simulink model "ACStesbed1"  (R2013b)
settings: Solver=ode45  StartTime=0.0  StopTime=10000  FixedStep=0.01  RelTol=1e-3
StartFcn:
  | InitializeModel
undefined symbols (not defined in the file or in its folder): DiscIntNeverNeededParam, e0_0, e1_0, e2_0, e3_0, magnitude, OrbData, params
libraries: aerolibutil x29, vrlib x26, satellite_control_lib x17, aerolibtransform2 x5, dspmtrx3 x5, aerolib6dofsys x4, dspinverses x3, simulink x3, aerolib6dof2 x1
(part 2 of 2)

== system ACStesbed1/CentralComputer/SatAttitude/BINS/OrbitalBasis ==
  vj2000 : Inport
  rj2000 : Inport  Port=2
  Cross Product : vrlib/Utilities/Cross Product
  Cross Product1 : vrlib/Utilities/Cross Product
  Direction Cosine Matrix to Quaternions : aerolibtransform2/Direction Cosine Matrix  to Quaternions
  Display4 : Display
  Divide : Product  Inputs=*/
  Gain : Gain  Gain=-1
  Matrix Concatenate : Concatenate  NumInputs=3  Mode=Multidimensional array  ConcatenateDimension=2
  Normalize Vector : vrlib/Utilities/Normalize Vector  maxzero=0.00001
  Normalize Vector1 : vrlib/Utilities/Normalize Vector  maxzero=0.00001
  Signal Specification : SignalSpecification  Dimensions=3
  Signal Specification1 : SignalSpecification  Dimensions=3
  Transpose1 : dspmtrx3/Transpose  Hermitian=off  overflowFlag=off
  vectnorm : Fcn  Expr=u(1)^2+u(2)^2+u(3)^2
  Qjo : Outport
  Worb_j : Outport  Port=2
  wires:
  Cross Product1/1 -> Signal Specification1/1  "iorb"
  Normalize Vector/1 -> Matrix Concatenate/2, Cross Product1/1  "jorb"
  Matrix Concatenate/1 -> Transpose1/1  "DCMoj"
  rj2000/1 -> Cross Product/2, Normalize Vector/1, vectnorm/1
  vj2000/1 -> Cross Product/1
  Direction Cosine Matrix to Quaternions/1 -> Display4/1, Qjo/1  "Qjo"
  Normalize Vector1/1 -> Matrix Concatenate/3, Cross Product1/2  "korb"
  Cross Product/1 -> Signal Specification/1
  Gain/1 -> Divide/1
  vectnorm/1 -> Divide/2
  Divide/1 -> Worb_j/1
  Signal Specification/1 -> Gain/1, Normalize Vector1/1
  Signal Specification1/1 -> Matrix Concatenate/1
  Transpose1/1 -> Direction Cosine Matrix to Quaternions/1  "DCMjo"

== system ACStesbed1/CentralComputer/SatAttitude/BINS/SIgnQuat ==
  Q : Inport
  Product : Product
  Selector2 : Selector  InputPortWidth=4  IndexOptions=Index vector (dialog)  Indices=[1]  OutputSizes=1
  Sign : Signum
  Q' : Outport
  wires:
  Q/1 -> Product/2, Selector2/1
  Product/1 -> Q'/1
  Sign/1 -> Product/1
  Selector2/1 -> Sign/1

== system ACStesbed1/CentralComputer/SatAttitude/BINS/SIgnQuat1 ==
  Q : Inport
  Constant : Constant
  Constant1 : Constant  Value=-1
  Product : Product
  Selector2 : Selector  InputPortWidth=4  IndexOptions=Index vector (dialog)  Indices=[1]  OutputSizes=1
  Switch : Switch
  Q' : Outport
  wires:
  Q/1 -> Product/2, Selector2/1
  Product/1 -> Q'/1
  Switch/1 -> Product/1
  Selector2/1 -> Switch/2
  Constant/1 -> Switch/1
  Constant1/1 -> Switch/3

== system ACStesbed1/CentralComputer/SatAttitude/BINS/SIgnQuat2 ==
  Q : Inport
  Constant : Constant
  Constant1 : Constant  Value=-1
  Product : Product
  Selector2 : Selector  InputPortWidth=4  IndexOptions=Index vector (dialog)  Indices=[1]  OutputSizes=1
  Switch : Switch
  Q' : Outport
  wires:
  Q/1 -> Product/2, Selector2/1
  Product/1 -> Q'/1
  Switch/1 -> Product/1
  Selector2/1 -> Switch/2
  Constant/1 -> Switch/1
  Constant1/1 -> Switch/3

== system ACStesbed1/CentralComputer/SatAttitude/BINS/SIgnQuat3 ==
  Q : Inport
  Constant : Constant
  Constant1 : Constant  Value=-1
  Product : Product
  Selector2 : Selector  InputPortWidth=4  IndexOptions=Index vector (dialog)  Indices=[1]  OutputSizes=1
  Switch : Switch
  Q' : Outport
  wires:
  Q/1 -> Product/2, Selector2/1
  Product/1 -> Q'/1
  Switch/1 -> Product/1
  Selector2/1 -> Switch/2
  Constant/1 -> Switch/1
  Constant1/1 -> Switch/3

== system ACStesbed1/CentralComputer/SatAttitude/BINS/SIgnQuat4 ==
  Q : Inport
  Constant : Constant
  Constant1 : Constant  Value=-1
  Product : Product
  Selector2 : Selector  InputPortWidth=4  IndexOptions=Index vector (dialog)  Indices=[1]  OutputSizes=1
  Switch : Switch
  Q' : Outport
  wires:
  Q/1 -> Product/2, Selector2/1
  Product/1 -> Q'/1
  Switch/1 -> Product/1
  Selector2/1 -> Switch/2
  Constant/1 -> Switch/1
  Constant1/1 -> Switch/3

== system ACStesbed1/CentralComputer/SatAttitude/BINS/quatint ==
  p q r : Inport
  q_init : Inport  Port=2
  q0 q1 q2 q3 : Integrator  InitialConditionSource=external  InitialCondition=[e0_0 e1_0 e2_0 e3_0]
  qdot : aerolib6dofsys/DCM & Euler Angles (Quaternion)/qdot
  q : Outport
  wires:
  q0 q1 q2 q3/1 -> q/1, qdot/2
  q_init/1 -> q0 q1 q2 q3/2
  p q r/1 -> qdot/1
  qdot/1 -> q0 q1 q2 q3/1

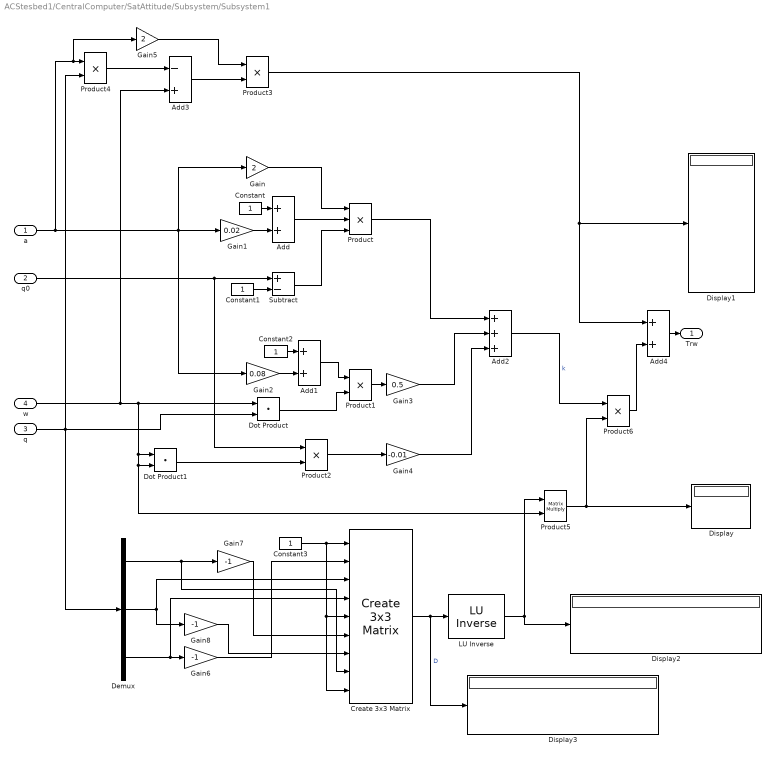
== system ACStesbed1/CentralComputer/SatAttitude/Subsystem/Subsystem1 ==
  a : Inport
  q0 : Inport  Port=2
  q : Inport  Port=3
  w : Inport  Port=4
  " LU Inverse" : dspinverses/ LU Inverse
  Add : Sum
  Add1 : Sum
  Add2 : Sum  Inputs=+++
  Add3 : Sum  Inputs=-+
  Add4 : Sum
  Constant{,1..3} (4 alike) : Constant
  Create 3x3 Matrix : aerolibutil/Create 3x3 Matrix
  Demux : Demux  Outputs=3
  Display{,1..3} (4 alike) : Display
  Dot Product : DotProduct  InputSameDT=on  OutDataTypeStr=Inherit: Inherit via internal rule
  Dot Product1 : DotProduct  InputSameDT=on  OutDataTypeStr=Inherit: Inherit via internal rule
  Gain : Gain  Gain=2
  Gain1 : Gain  Gain=0.02
  Gain2 : Gain  Gain=0.08
  Gain3 : Gain  Gain=0.5
  Gain4 : Gain  Gain=-0.01
  Gain5 : Gain  Gain=2
  Gain6 : Gain  Gain=-1
  Gain7 : Gain  Gain=-1
  Gain8 : Gain  Gain=-1
  Product : Product  Inputs=3
  Product{1..4,6} (5 alike) : Product
  Product5 : Product  Multiplication=Matrix(*)
  Subtract : Sum  Inputs=+-
  Trw : Outport
  wires:
  Gain1/1 -> Add/2
  Constant/1 -> Add/1
  a/1 -> Gain5/1, Product4/1, Gain2/1, Gain/1, Gain1/1
  Constant1/1 -> Subtract/2
  q0/1 -> Product2/1, Subtract/1
  Gain/1 -> Product/1
  Add/1 -> Product/2
  Subtract/1 -> Product/3
  w/1 -> Add3/2, Dot Product/1, Product5/2, Dot Product1/2, Dot Product1/1
  q/1 -> Demux/1, Product4/2, Dot Product/2
  Gain2/1 -> Add1/2
  Constant2/1 -> Add1/1
  Add1/1 -> Product1/1
  Dot Product/1 -> Product1/2
  Product1/1 -> Gain3/1
  Dot Product1/1 -> Product2/2
  Product2/1 -> Gain4/1
  Product/1 -> Add2/1
  Gain3/1 -> Add2/2
  Gain4/1 -> Add2/3
  Add2/1 -> Product6/1  "k"
  Product4/1 -> Add3/1
  Gain5/1 -> Product3/1
  Add3/1 -> Product3/2
  Constant3/1 -> Create 3x3 Matrix/9, Create 3x3 Matrix/5, Create 3x3 Matrix/1
  Demux/3 -> Create 3x3 Matrix/4, Gain6/1
  Gain6/1 -> Create 3x3 Matrix/2
  Demux/2 -> Gain8/1, Create 3x3 Matrix/3
  Demux/1 -> Create 3x3 Matrix/8, Gain7/1
  Gain7/1 -> Create 3x3 Matrix/6
  Gain8/1 -> Create 3x3 Matrix/7
  Create 3x3 Matrix/1 -> Display3/1, " LU Inverse"/1  "D"
  " LU Inverse"/1 -> Product5/1, Display2/1
  Product5/1 -> Display/1, Product6/2
  Add4/1 -> Trw/1
  Product6/1 -> Add4/2
  Product3/1 -> Display1/1, Add4/1

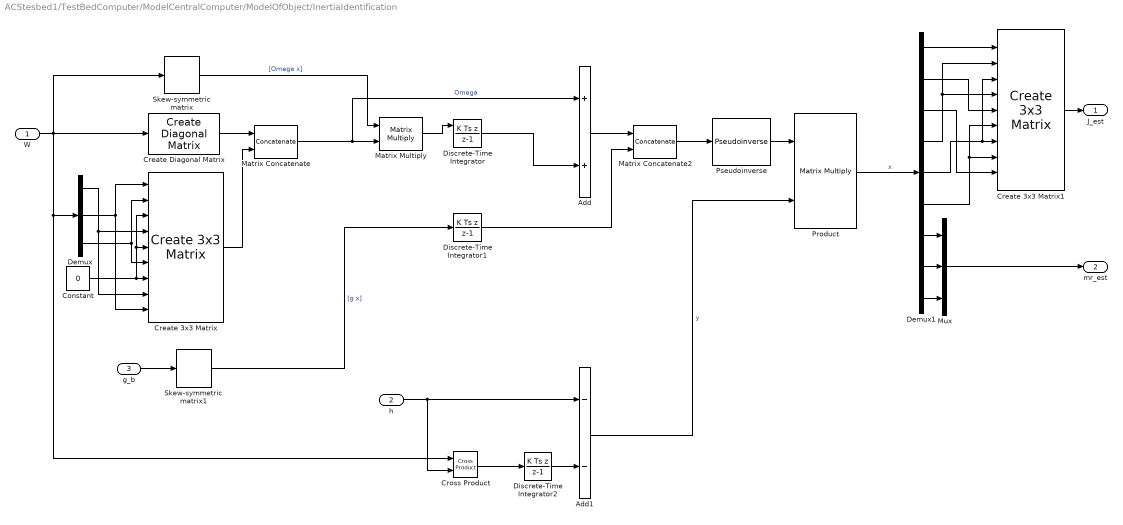
== system ACStesbed1/TestBedComputer/ModelCentralComputer/ModelOfObject/InertiaIdentification ==
  W : Inport
  h : Inport  Port=2
  g_b : Inport  Port=3
  Add : Sum
  Add1 : Sum  Inputs=--
  Constant : Constant  Value=0
  Create 3x3 Matrix : aerolibutil/Create 3x3 Matrix
  Create 3x3 Matrix1 : aerolibutil/Create 3x3 Matrix
  Create Diagonal Matrix : dspmtrx3/Create Diagonal Matrix
  Cross Product : vrlib/Utilities/Cross Product
  Demux : Demux  Outputs=3
  Demux1 : Demux  Outputs=9
  Discrete-Time Integrator : DiscreteIntegrator  IntegratorMethod=Integration: Backward Euler  InitialConditionSource=external  ICPrevOutput=DiscIntNeverNeededParam  ICPrevScaledInput=DiscIntNeverNeededParam
  Discrete-Time Integrator1 : DiscreteIntegrator  IntegratorMethod=Integration: Backward Euler  ICPrevOutput=DiscIntNeverNeededParam  ICPrevScaledInput=DiscIntNeverNeededParam
  Discrete-Time Integrator2 : DiscreteIntegrator  IntegratorMethod=Integration: Backward Euler  ICPrevOutput=DiscIntNeverNeededParam  ICPrevScaledInput=DiscIntNeverNeededParam
  Matrix Concatenate : Concatenate  Mode=Multidimensional array  ConcatenateDimension=2
  Matrix Concatenate2 : Concatenate  Mode=Multidimensional array  ConcatenateDimension=2
  Matrix Multiply : Product  Multiplication=Matrix(*)
  Mux : Mux  Inputs=3
  Product : Product  Multiplication=Matrix(*)
  Pseudoinverse : dspinverses/Pseudoinverse  wanterr=off
  Skew-symmetric matrix : satellite_control_lib/Skew-symmetric matrix
  Skew-symmetric matrix1 : satellite_control_lib/Skew-symmetric matrix
  J_est : Outport
  mr_est : Outport  Port=2
  wires:
  Product/1 -> Demux1/1  "x"
  Pseudoinverse/1 -> Product/1
  Add1/1 -> Product/2  "y"
  W/1 -> Skew-symmetric matrix/1, Demux/1, Cross Product/1, Create Diagonal Matrix/1
  Demux/2 -> Create 3x3 Matrix/9, Create 3x3 Matrix/1
  Demux/3 -> Create 3x3 Matrix/6, Create 3x3 Matrix/2
  Demux/1 -> Create 3x3 Matrix/8, Create 3x3 Matrix/4
  Constant/1 -> Create 3x3 Matrix/3, Create 3x3 Matrix/5, Create 3x3 Matrix/7
  Create Diagonal Matrix/1 -> Matrix Concatenate/1
  Create 3x3 Matrix/1 -> Matrix Concatenate/2
  Matrix Concatenate/1 -> Add/1, Matrix Multiply/2  "Omega"
  Skew-symmetric matrix/1 -> Matrix Multiply/1  "[Omega x]"
  g_b/1 -> Skew-symmetric matrix1/1
  Skew-symmetric matrix1/1 -> Discrete-Time Integrator1/1  "[g x]"
  Matrix Multiply/1 -> Discrete-Time Integrator/1
  Discrete-Time Integrator1/1 -> Matrix Concatenate2/2
  Discrete-Time Integrator/1 -> Add/2
  Add/1 -> Matrix Concatenate2/1
  h/1 -> Cross Product/2, Add1/1
  Discrete-Time Integrator2/1 -> Add1/2
  Cross Product/1 -> Discrete-Time Integrator2/1
  Demux1/1 -> Create 3x3 Matrix1/1
  Demux1/2 -> Create 3x3 Matrix1/5
  Demux1/3 -> Create 3x3 Matrix1/9
  Demux1/4 -> Create 3x3 Matrix1/4, Create 3x3 Matrix1/2
  Demux1/5 -> Create 3x3 Matrix1/7, Create 3x3 Matrix1/3
  Demux1/6 -> Create 3x3 Matrix1/8, Create 3x3 Matrix1/6
  Create 3x3 Matrix1/1 -> J_est/1
  Demux1/7 -> Mux/1
  Demux1/9 -> Mux/3
  Demux1/8 -> Mux/2
  Mux/1 -> mr_est/1
  Matrix Concatenate2/1 -> Pseudoinverse/1

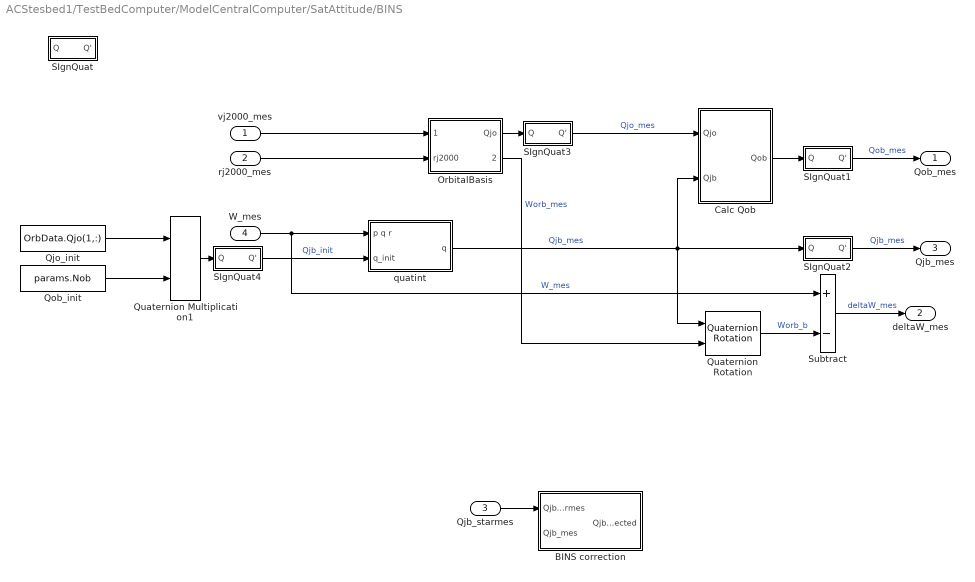
== system ACStesbed1/TestBedComputer/ModelCentralComputer/SatAttitude/BINS ==
  vj2000_mes : Inport
  rj2000_mes : Inport  Port=2
  Qjb_starmes : Inport  Port=3
  W_mes : Inport  Port=4
  BINS correction : Subsystem
  Calc Qob : Subsystem
  OrbitalBasis : Subsystem
  Qjo_init : Constant  Value=OrbData.Qjo(1,:)
  Qob_init : Constant  Value=params.Nob
  Quaternion Multiplication1 : aerolibutil/Quaternion Multiplication
  Quaternion Rotation : aerolibutil/Quaternion Rotation
  SIgnQuat : Subsystem
  SIgnQuat1 : Subsystem
  SIgnQuat2 : Subsystem
  SIgnQuat3 : Subsystem
  SIgnQuat4 : Subsystem
  Subtract : Sum  Inputs=+-
  quatint : Subsystem
  Qob_mes : Outport
  deltaW_mes : Outport  Port=2
  Qjb_mes : Outport  Port=3
  wires:
  Qjb_starmes/1 -> BINS correction/1(Qjb_starmes)
  quatint/1(q) -> SIgnQuat2/1(Q), Calc Qob/2(Qjb), Quaternion Rotation/1  "Qjb_mes"
  Calc Qob/1(Qob) -> SIgnQuat1/1(Q)
  rj2000_mes/1 -> OrbitalBasis/2(rj2000)
  vj2000_mes/1 -> OrbitalBasis/1(vj2000)
  OrbitalBasis/1(Qjo) -> SIgnQuat3/1(Q)
  OrbitalBasis/2(Worb_j) -> Quaternion Rotation/2  "Worb_mes"
  W_mes/1 -> Subtract/1, quatint/1(p q r)  "W_mes"
  Subtract/1 -> deltaW_mes/1  "deltaW_mes"
  Qjo_init/1 -> Quaternion Multiplication1/1
  Qob_init/1 -> Quaternion Multiplication1/2
  Quaternion Multiplication1/1 -> SIgnQuat4/1(Q)
  Quaternion Rotation/1 -> Subtract/2  "Worb_b"
  SIgnQuat1/1(Q') -> Qob_mes/1  "Qob_mes"
  SIgnQuat2/1(Q') -> Qjb_mes/1  "Qjb_mes"
  SIgnQuat3/1(Q') -> Calc Qob/1(Qjo)  "Qjo_mes"
  SIgnQuat4/1(Q') -> quatint/2(q_init)  "Qjb_init"

== system ACStesbed1/TestBedComputer/ModelCentralComputer/SatAttitude/Subsystem ==
  In1 : Inport
  In2 : Inport  Port=2
  In3 : Inport  Port=3
  Gain : Gain  Gain=-1
  Product5 : Product  Multiplication=Matrix(*)
  Selector : Selector  InputPortWidth=4  IndexOptions=Index vector (dialog)  Indices=1  OutputSizes=1
  Selector1 : Selector  InputPortWidth=4  IndexOptions=Index vector (dialog)  Indices=[2 3 4]  OutputSizes=1
  Subsystem1 : Subsystem
  a : Constant  Value=-0.9
  Out1 : Outport
  wires:
  Subsystem1/1(Trw) -> Product5/2
  Selector1/1 -> Subsystem1/3(q)
  a/1 -> Subsystem1/1(a)
  Selector/1 -> Subsystem1/2(q0)  "1"
  Product5/1 -> Gain/1
  In2/1 -> Selector1/1, Selector/1
  In3/1 -> Subsystem1/4(w)
  In1/1 -> Product5/1
  Gain/1 -> Out1/1

== system ACStesbed1/TestBedComputer/ModelObject/Inertia/deltaJ1 ==
  d : Inport
  e : Inport  Port=2
  rho : Inport  Port=3
  Add : Sum  Inputs=3
  Constant : Constant  Value=params.bmass
  Gain : Gain  Gain=-1
  Math Function : Math  Operator=magnitude^2  SaturateOnIntegerOverflow=on
  Product{,4..6} (4 alike) : Product
  Product1 : Product  Multiplication=Matrix(*)
  Product2 : Product  Multiplication=Matrix(*)
  Product3 : Product  Multiplication=Matrix(*)
  Skew-symmetric matrix : satellite_control_lib/Skew-symmetric matrix
  Skew-symmetric matrix1 : satellite_control_lib/Skew-symmetric matrix
  deltaJ : Outport
  wires:
  Constant/1 -> Gain/1
  e/1 -> Skew-symmetric matrix/1
  rho/1 -> Skew-symmetric matrix1/1
  Product/1 -> deltaJ/1  "(-m)(d^2[e x]^2+d[rho x][e x]+d[e x][rho x])"
  Gain/1 -> Product/1
  d/1 -> Math Function/1, Product6/1, Product5/1
  Skew-symmetric matrix/1 -> Product2/2, Product3/1, Product1/1, Product1/2  "[e x]"
  Math Function/1 -> Product4/1
  Product1/1 -> Product4/2
  Skew-symmetric matrix1/1 -> Product3/2, Product2/1  "[rho x]"
  Product3/1 -> Product5/2
  Product2/1 -> Product6/2
  Add/1 -> Product/2
  Product4/1 -> Add/1
  Product5/1 -> Add/2
  Product6/1 -> Add/3

== system ACStesbed1/TestBedComputer/ModelObject/Inertia/deltaJ2 ==
  d : Inport
  e : Inport  Port=2
  rho : Inport  Port=3
  Add : Sum  Inputs=3
  Constant : Constant  Value=params.bmass
  Gain : Gain  Gain=-1
  Math Function : Math  Operator=magnitude^2  SaturateOnIntegerOverflow=on
  Product{,4..6} (4 alike) : Product
  Product1 : Product  Multiplication=Matrix(*)
  Product2 : Product  Multiplication=Matrix(*)
  Product3 : Product  Multiplication=Matrix(*)
  Skew-symmetric matrix : satellite_control_lib/Skew-symmetric matrix
  Skew-symmetric matrix1 : satellite_control_lib/Skew-symmetric matrix
  deltaJ : Outport
  wires:
  Product6/1 -> Add/3
  Product5/1 -> Add/2
  Product4/1 -> Add/1
  Add/1 -> Product/2
  Product2/1 -> Product6/2
  Product3/1 -> Product5/2
  Skew-symmetric matrix1/1 -> Product2/1, Product3/2  "[rho x]"
  Product1/1 -> Product4/2
  Math Function/1 -> Product4/1
  Skew-symmetric matrix/1 -> Product1/2, Product1/1, Product3/1, Product2/2  "[e x]"
  d/1 -> Product5/1, Product6/1, Math Function/1
  Gain/1 -> Product/1
  Product/1 -> deltaJ/1  "(-m)(d^2[e x]^2+d[rho x][e x]+d[e x][rho x])"
  rho/1 -> Skew-symmetric matrix1/1
  e/1 -> Skew-symmetric matrix/1
  Constant/1 -> Gain/1

== system ACStesbed1/TestBedComputer/ModelObject/Inertia/deltaJ3 ==
  d : Inport
  e : Inport  Port=2
  rho : Inport  Port=3
  Add : Sum  Inputs=3
  Constant : Constant  Value=params.bmass
  Gain : Gain  Gain=-1
  Math Function : Math  Operator=magnitude^2  SaturateOnIntegerOverflow=on
  Product{,4..6} (4 alike) : Product
  Product1 : Product  Multiplication=Matrix(*)
  Product2 : Product  Multiplication=Matrix(*)
  Product3 : Product  Multiplication=Matrix(*)
  Skew-symmetric matrix : satellite_control_lib/Skew-symmetric matrix
  Skew-symmetric matrix1 : satellite_control_lib/Skew-symmetric matrix
  deltaJ : Outport
  wires:
  Constant/1 -> Gain/1
  e/1 -> Skew-symmetric matrix/1
  rho/1 -> Skew-symmetric matrix1/1
  Product/1 -> deltaJ/1  "(-m)(d^2[e x]^2+d[rho x][e x]+d[e x][rho x])"
  Gain/1 -> Product/1
  d/1 -> Math Function/1, Product6/1, Product5/1
  Skew-symmetric matrix/1 -> Product2/2, Product3/1, Product1/1, Product1/2  "[e x]"
  Math Function/1 -> Product4/1
  Product1/1 -> Product4/2
  Skew-symmetric matrix1/1 -> Product3/2, Product2/1  "[rho x]"
  Product3/1 -> Product5/2
  Product2/1 -> Product6/2
  Add/1 -> Product/2
  Product4/1 -> Add/1
  Product5/1 -> Add/2
  Product6/1 -> Add/3

== system ACStesbed1/TestBedComputer/ModelObject/TestBedDynamics/quatint ==
  p q r : Inport
  q_init : Inport  Port=2
  Discrete-Time Integrator : DiscreteIntegrator  InitialConditionSource=external  ICPrevOutput=DiscIntNeverNeededParam  ICPrevScaledInput=DiscIntNeverNeededParam
  qdot : aerolib6dofsys/DCM & Euler Angles (Quaternion)/qdot
  q : Outport
  wires:
  Discrete-Time Integrator/1 -> q/1, qdot/2
  q_init/1 -> Discrete-Time Integrator/2
  p q r/1 -> qdot/1
  qdot/1 -> Discrete-Time Integrator/1

== system ACStesbed1/TestBedComputer/ModelObject/Torques/Tm ==
  L : Inport
  B : Inport  Port=2
  Ldisturb : Inport  Port=3
  Tm : Outport
  wires:
  L/1 -> Tm/1

== system ACStesbed1/TestBedComputer/ModelObject/Torques/Tothers ==
  Something : Inport
  Tothers : Outport
  wires:
  Something/1 -> Tothers/1

== system ACStesbed1/TestBedComputer/ModelObject/Torques/Trw ==
  dh : Inport
  W : Inport  Port=2
  h : Inport  Port=3
  Add : Sum
  Cross Product : vrlib/Utilities/Cross Product
  Gain : Gain  Gain=-1
  Trw : Outport
  wires:
  W/1 -> Cross Product/1
  Gain/1 -> Trw/1  "Trw"
  Cross Product/1 -> Add/2  "Wxh"
  Add/1 -> Gain/1  "(dH+WxH)"
  dh/1 -> Add/1
  h/1 -> Cross Product/2

== system ACStesbed1/TestBedComputer/ModelCentralComputer/SatAttitude/BINS/BINS correction ==
  Qjb_starmes : Inport
  Qjb_mes : Inport  Port=2
  Quaternion Conjugate : aerolibutil/Quaternion Conjugate
  Quaternion Conjugate1 : aerolibutil/Quaternion Conjugate
  Quaternion Multiplication : aerolibutil/Quaternion Multiplication
  Quaternion Multiplication1 : aerolibutil/Quaternion Multiplication
  Qjb_corrected : Outport
  wires:
  Quaternion Multiplication1/1 -> Qjb_corrected/1  "Qjb_corrected"
  Quaternion Conjugate1/1 -> Quaternion Multiplication1/1
  Qjb_mes/1 -> Quaternion Multiplication1/2, Quaternion Multiplication/2
  Quaternion Multiplication/1 -> Quaternion Conjugate1/1  "Nbb_mes"
  Qjb_starmes/1 -> Quaternion Conjugate/1
  Quaternion Conjugate/1 -> Quaternion Multiplication/1  "conjQjb_starmes"

== system ACStesbed1/TestBedComputer/ModelCentralComputer/SatAttitude/BINS/Calc Qob ==
  Qjo : Inport
  Qjb : Inport  Port=2
  Quaternion Inverse : aerolibutil/Quaternion Inverse
  Quaternion Multiplication : aerolibutil/Quaternion Multiplication
  Qob : Outport
  wires:
  Qjb/1 -> Quaternion Multiplication/2  "Qjb"
  Qjo/1 -> Quaternion Inverse/1  "Qjo"
  Quaternion Inverse/1 -> Quaternion Multiplication/1
  Quaternion Multiplication/1 -> Qob/1

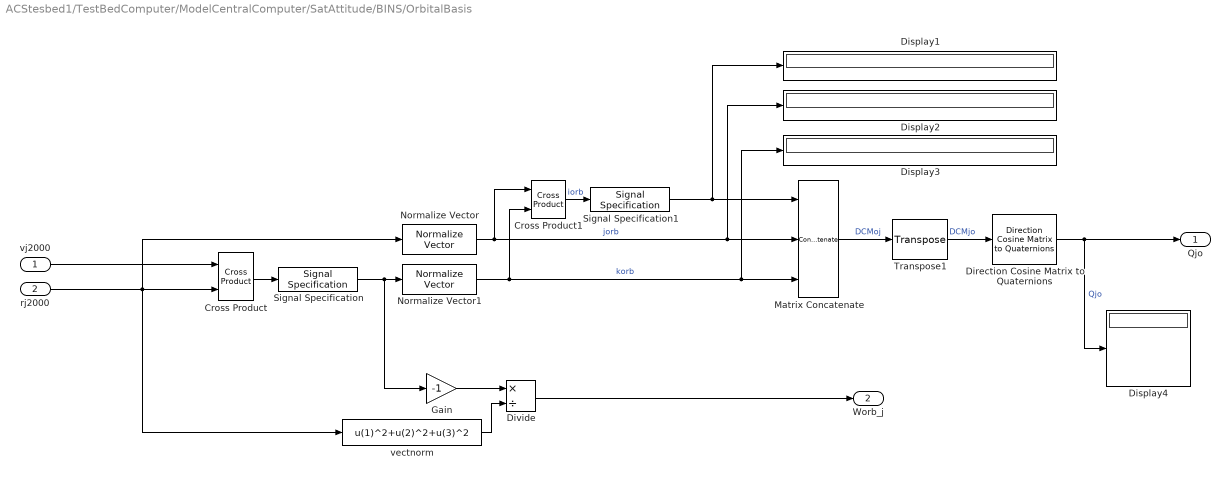
== system ACStesbed1/TestBedComputer/ModelCentralComputer/SatAttitude/BINS/OrbitalBasis ==
  vj2000 : Inport
  rj2000 : Inport  Port=2
  Cross Product : vrlib/Utilities/Cross Product
  Cross Product1 : vrlib/Utilities/Cross Product
  Direction Cosine Matrix to Quaternions : aerolibtransform2/Direction Cosine Matrix  to Quaternions
  Display{1..4} (4 alike) : Display
  Divide : Product  Inputs=*/
  Gain : Gain  Gain=-1
  Matrix Concatenate : Concatenate  NumInputs=3  Mode=Multidimensional array  ConcatenateDimension=2
  Normalize Vector : vrlib/Utilities/Normalize Vector  maxzero=0.00001
  Normalize Vector1 : vrlib/Utilities/Normalize Vector  maxzero=0.00001
  Signal Specification : SignalSpecification  Dimensions=3
  Signal Specification1 : SignalSpecification  Dimensions=3
  Transpose1 : dspmtrx3/Transpose  Hermitian=off  overflowFlag=off
  vectnorm : Fcn  Expr=u(1)^2+u(2)^2+u(3)^2
  Qjo : Outport
  Worb_j : Outport  Port=2
  wires:
  Cross Product1/1 -> Signal Specification1/1  "iorb"
  Normalize Vector/1 -> Display2/1, Matrix Concatenate/2, Cross Product1/1  "jorb"
  Matrix Concatenate/1 -> Transpose1/1  "DCMoj"
  rj2000/1 -> Cross Product/2, Normalize Vector/1, vectnorm/1
  vj2000/1 -> Cross Product/1
  Direction Cosine Matrix to Quaternions/1 -> Display4/1, Qjo/1  "Qjo"
  Normalize Vector1/1 -> Display3/1, Matrix Concatenate/3, Cross Product1/2  "korb"
  Cross Product/1 -> Signal Specification/1
  Gain/1 -> Divide/1
  vectnorm/1 -> Divide/2
  Divide/1 -> Worb_j/1
  Signal Specification/1 -> Gain/1, Normalize Vector1/1
  Signal Specification1/1 -> Display1/1, Matrix Concatenate/1
  Transpose1/1 -> Direction Cosine Matrix to Quaternions/1  "DCMjo"

== system ACStesbed1/TestBedComputer/ModelCentralComputer/SatAttitude/BINS/SIgnQuat ==
  Q : Inport
  Product : Product
  Selector2 : Selector  InputPortWidth=4  IndexOptions=Index vector (dialog)  Indices=[1]  OutputSizes=1
  Sign : Signum
  Q' : Outport
  wires:
  Q/1 -> Product/2, Selector2/1
  Product/1 -> Q'/1
  Sign/1 -> Product/1
  Selector2/1 -> Sign/1

== system ACStesbed1/TestBedComputer/ModelCentralComputer/SatAttitude/BINS/SIgnQuat1 ==
  Q : Inport
  Constant : Constant
  Constant1 : Constant  Value=-1
  Product : Product
  Selector2 : Selector  InputPortWidth=4  IndexOptions=Index vector (dialog)  Indices=[1]  OutputSizes=1
  Switch : Switch
  Q' : Outport
  wires:
  Q/1 -> Product/2, Selector2/1
  Product/1 -> Q'/1
  Switch/1 -> Product/1
  Selector2/1 -> Switch/2
  Constant/1 -> Switch/1
  Constant1/1 -> Switch/3

== system ACStesbed1/TestBedComputer/ModelCentralComputer/SatAttitude/BINS/SIgnQuat2 ==
  Q : Inport
  Constant : Constant
  Constant1 : Constant  Value=-1
  Product : Product
  Selector2 : Selector  InputPortWidth=4  IndexOptions=Index vector (dialog)  Indices=[1]  OutputSizes=1
  Switch : Switch
  Q' : Outport
  wires:
  Q/1 -> Product/2, Selector2/1
  Product/1 -> Q'/1
  Switch/1 -> Product/1
  Selector2/1 -> Switch/2
  Constant/1 -> Switch/1
  Constant1/1 -> Switch/3

== system ACStesbed1/TestBedComputer/ModelCentralComputer/SatAttitude/BINS/SIgnQuat3 ==
  Q : Inport
  Constant : Constant
  Constant1 : Constant  Value=-1
  Product : Product
  Selector2 : Selector  InputPortWidth=4  IndexOptions=Index vector (dialog)  Indices=[1]  OutputSizes=1
  Switch : Switch
  Q' : Outport
  wires:
  Q/1 -> Product/2, Selector2/1
  Product/1 -> Q'/1
  Switch/1 -> Product/1
  Selector2/1 -> Switch/2
  Constant/1 -> Switch/1
  Constant1/1 -> Switch/3

== system ACStesbed1/TestBedComputer/ModelCentralComputer/SatAttitude/BINS/SIgnQuat4 ==
  Q : Inport
  Constant : Constant
  Constant1 : Constant  Value=-1
  Product : Product
  Selector2 : Selector  InputPortWidth=4  IndexOptions=Index vector (dialog)  Indices=[1]  OutputSizes=1
  Switch : Switch
  Q' : Outport
  wires:
  Q/1 -> Product/2, Selector2/1
  Product/1 -> Q'/1
  Switch/1 -> Product/1
  Selector2/1 -> Switch/2
  Constant/1 -> Switch/1
  Constant1/1 -> Switch/3

== system ACStesbed1/TestBedComputer/ModelCentralComputer/SatAttitude/BINS/quatint ==
  p q r : Inport
  q_init : Inport  Port=2
  q0 q1 q2 q3 : Integrator  InitialConditionSource=external  InitialCondition=[e0_0 e1_0 e2_0 e3_0]
  qdot : aerolib6dofsys/DCM & Euler Angles (Quaternion)/qdot
  q : Outport
  wires:
  q0 q1 q2 q3/1 -> q/1, qdot/2
  q_init/1 -> q0 q1 q2 q3/2
  p q r/1 -> qdot/1
  qdot/1 -> q0 q1 q2 q3/1

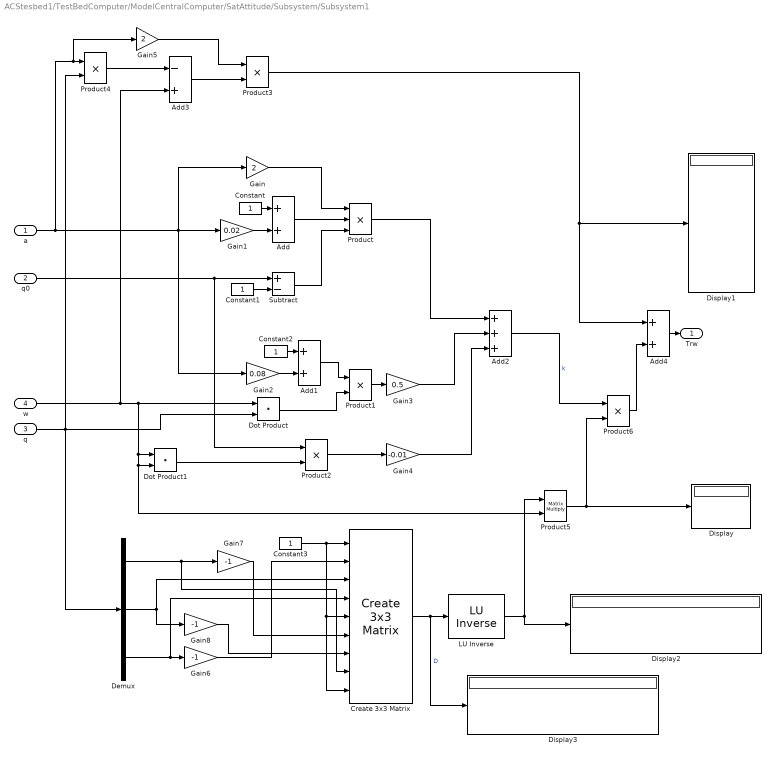
== system ACStesbed1/TestBedComputer/ModelCentralComputer/SatAttitude/Subsystem/Subsystem1 ==
  a : Inport
  q0 : Inport  Port=2
  q : Inport  Port=3
  w : Inport  Port=4
  " LU Inverse" : dspinverses/ LU Inverse
  Add : Sum
  Add1 : Sum
  Add2 : Sum  Inputs=+++
  Add3 : Sum  Inputs=-+
  Add4 : Sum
  Constant{,1..3} (4 alike) : Constant
  Create 3x3 Matrix : aerolibutil/Create 3x3 Matrix
  Demux : Demux  Outputs=3
  Display{,1..3} (4 alike) : Display
  Dot Product : DotProduct  InputSameDT=on  OutDataTypeStr=Inherit: Inherit via internal rule
  Dot Product1 : DotProduct  InputSameDT=on  OutDataTypeStr=Inherit: Inherit via internal rule
  Gain : Gain  Gain=2
  Gain1 : Gain  Gain=0.02
  Gain2 : Gain  Gain=0.08
  Gain3 : Gain  Gain=0.5
  Gain4 : Gain  Gain=-0.01
  Gain5 : Gain  Gain=2
  Gain6 : Gain  Gain=-1
  Gain7 : Gain  Gain=-1
  Gain8 : Gain  Gain=-1
  Product : Product  Inputs=3
  Product{1..4,6} (5 alike) : Product
  Product5 : Product  Multiplication=Matrix(*)
  Subtract : Sum  Inputs=+-
  Trw : Outport
  wires:
  Gain1/1 -> Add/2
  Constant/1 -> Add/1
  a/1 -> Gain5/1, Product4/1, Gain2/1, Gain/1, Gain1/1
  Constant1/1 -> Subtract/2
  q0/1 -> Product2/1, Subtract/1
  Gain/1 -> Product/1
  Add/1 -> Product/2
  Subtract/1 -> Product/3
  w/1 -> Add3/2, Dot Product/1, Product5/2, Dot Product1/2, Dot Product1/1
  q/1 -> Demux/1, Product4/2, Dot Product/2
  Gain2/1 -> Add1/2
  Constant2/1 -> Add1/1
  Add1/1 -> Product1/1
  Dot Product/1 -> Product1/2
  Product1/1 -> Gain3/1
  Dot Product1/1 -> Product2/2
  Product2/1 -> Gain4/1
  Product/1 -> Add2/1
  Gain3/1 -> Add2/2
  Gain4/1 -> Add2/3
  Add2/1 -> Product6/1  "k"
  Product4/1 -> Add3/1
  Gain5/1 -> Product3/1
  Add3/1 -> Product3/2
  Constant3/1 -> Create 3x3 Matrix/9, Create 3x3 Matrix/5, Create 3x3 Matrix/1
  Demux/3 -> Create 3x3 Matrix/4, Gain6/1
  Gain6/1 -> Create 3x3 Matrix/2
  Demux/2 -> Gain8/1, Create 3x3 Matrix/3
  Demux/1 -> Create 3x3 Matrix/8, Gain7/1
  Gain7/1 -> Create 3x3 Matrix/6
  Gain8/1 -> Create 3x3 Matrix/7
  Create 3x3 Matrix/1 -> Display3/1, " LU Inverse"/1  "D"
  " LU Inverse"/1 -> Product5/1, Display2/1
  Product5/1 -> Display/1, Product6/2
  Add4/1 -> Trw/1
  Product6/1 -> Add4/2
  Product3/1 -> Display1/1, Add4/1
